simulink model "mixer_test"  (Simulink 7.0)
settings: Solver=VariableStepDiscrete  StartTime=0.0  StopTime=1500  RelTol=1e-3
libraries: xbsIndex_r4 x28, simulink x8, casper_library x6
settings Model: Creator=User  LastModifiedBy=User

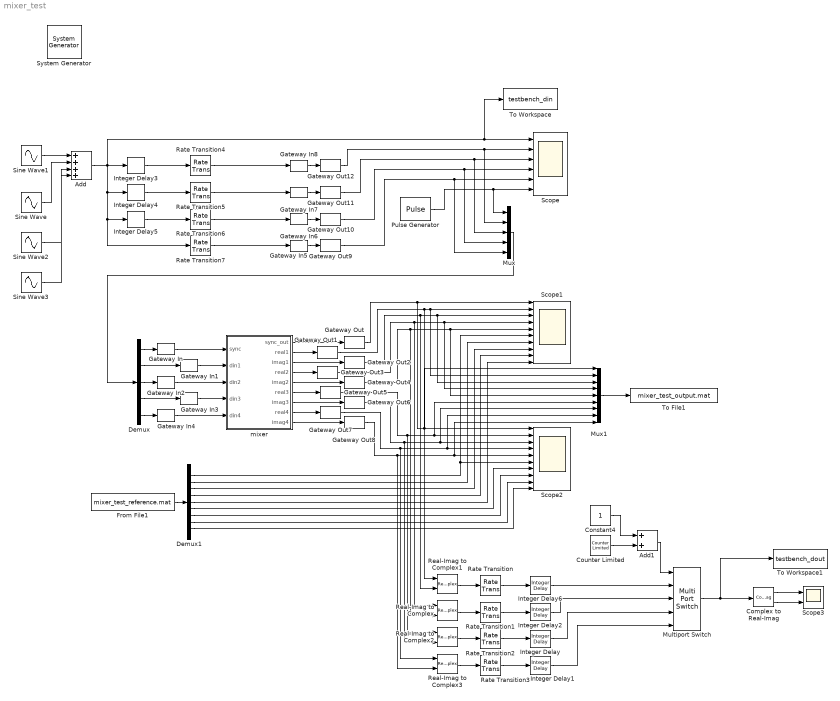
== system mixer_test ==
  " System Generator" : xbsIndex_r4/ System Generator  Tag=genX  SystemSampleTime=-1  xilinxfamily=Virtex4  part=xc4vsx35  speed=-10  package=ff668  synthesis_tool=XST  clock_wrapper=Clock Enables  directory=./netlist  testbench=off  simulink_period=1  sysclk_period=100  dcm_input_clock_period=100  incr_netlist=off  trim_vbits=Everywhere in SubSystem  dbl_ovrd=According to Block Masks  core_generation=According to Block Masks  run_coregen=off  deprecated_control=off  eval_field=0  block_type=sysgen
      settings: block_version=10.1.1
  Add : Sum  Inputs=++++  OutDataType=sfix(16)  OutScaling=2^-10
  Add1 : Sum  OutDataType=sfix(16)  OutScaling=2^-10
  Complex to Real-Imag : ComplexToRealImag
  Constant4 : Constant  OutDataType=sfix(16)  OutScaling=2^0
  Counter Limited : simulink/Sources/Counter Limited  SystemSampleTime=-1  uplimit=3  tsamp=-1
  Demux : Demux  Outputs=5
  Demux1 : Demux  Outputs=9
  From File1 : FromFile  FileName=mixer_test_reference.mat  SampleTime=1
  Gateway In : xbsIndex_r4/Gateway In  arith_type=Boolean  n_bits=16  bin_pt=14  quantization="Round  (unbiased: +/- Inf)"  overflow=Saturate  period=1  dbl_ovrd=off  timing_constraint=None  locs_specified=off  LOCs={}  block_type=gatewayin
      settings: infoedit="Gateway in block.  Converts inputs of type Simulink integer, double and fixed point to  Xilinx fixed point type.<P><P>Hardware notes:  In hardware these blocks become top level input ports."  block_version=10.1.1
  Gateway In{1..4,8} (5 alike) : xbsIndex_r4/Gateway In  arith_type="Signed  (2's comp)"  n_bits=16  bin_pt=13  quantization=Truncate  overflow=Wrap  period=1  dbl_ovrd=off  timing_constraint=None  locs_specified=off  LOCs={}  block_type=gatewayin
      settings: infoedit="Gateway in block.  Converts inputs of type Simulink integer, double and fixed point to  Xilinx fixed point type.<P><P>Hardware notes:  In hardware these blocks become top level input ports."  block_version=10.1.1
  Gateway In5 : xbsIndex_r4/Gateway In  arith_type="Signed  (2's comp)"  n_bits=16  bin_pt=13  quantization="Round  (unbiased: +/- Inf)"  overflow=Saturate  period=1  dbl_ovrd=off  timing_constraint=None  locs_specified=off  LOCs={}  block_type=gatewayin
      settings: infoedit="Gateway in block.  Converts inputs of type Simulink integer, double and fixed point to  Xilinx fixed point type.<P><P>Hardware notes:  In hardware these blocks become top level input ports."  block_version=10.1.1
  Gateway In6 : xbsIndex_r4/Gateway In  arith_type="Signed  (2's comp)"  n_bits=16  bin_pt=13  quantization="Round  (unbiased: +/- Inf)"  overflow=Saturate  period=1  dbl_ovrd=off  timing_constraint=None  locs_specified=off  LOCs={}  block_type=gatewayin
      settings: infoedit="Gateway in block.  Converts inputs of type Simulink integer, double and fixed point to  Xilinx fixed point type.<P><P>Hardware notes:  In hardware these blocks become top level input ports."  block_version=10.1.1
  Gateway In7 : xbsIndex_r4/Gateway In  arith_type="Signed  (2's comp)"  n_bits=16  bin_pt=13  quantization="Round  (unbiased: +/- Inf)"  overflow=Saturate  period=1  dbl_ovrd=off  timing_constraint=None  locs_specified=off  LOCs={}  block_type=gatewayin
      settings: infoedit="Gateway in block.  Converts inputs of type Simulink integer, double and fixed point to  Xilinx fixed point type.<P><P>Hardware notes:  In hardware these blocks become top level input ports."  block_version=10.1.1
  Gateway Out{,1..12} (13 alike) : xbsIndex_r4/Gateway Out  hdl_port=on  timing_constraint=None  locs_specified=off  LOCs={}  block_type=gatewayout
      settings: infoedit="Gateway out block.  Converts Xilinx fixed point inputs into ouputs of type Simulink integer, double, or fixed point.<P><P>Hardware notes:  In hardware these blocks become top level output ports or are discarded, depending on how they are configured."  block_version=10.1.1
  Integer Delay : simulink/Discrete/Integer Delay  vinit=0.0  samptime=0.25  NumDelays=3
  Integer Delay1 : simulink/Discrete/Integer Delay  vinit=0.0  samptime=0.25  NumDelays=4
  Integer Delay2 : simulink/Discrete/Integer Delay  vinit=0.0  samptime=0.25  NumDelays=2
  Integer Delay3 : simulink/Discrete/Integer Delay  vinit=0.0  samptime=-1  NumDelays=3
  Integer Delay4 : simulink/Discrete/Integer Delay  vinit=0.0  samptime=-1  NumDelays=2
  Integer Delay5 : simulink/Discrete/Integer Delay  vinit=0.0  samptime=-1  NumDelays=1
  Integer Delay6 : simulink/Discrete/Integer Delay  vinit=0.0  samptime=0.25  NumDelays=1
  Multiport Switch : MultiPortSwitch  OutDataType=sfix(16)  OutScaling=2^0
  Mux : Mux  Inputs=5
  Mux1 : Mux  Inputs=9
  Pulse Generator : DiscretePulseGenerator  Period=128  PhaseDelay=15
  Rate Transition{,1..7} (8 alike) : RateTransition
  Real-Imag to Complex{,1..3} (4 alike) : RealImagToComplex
  Scope : Scope  NumInputPorts=6
      settings: YMin=-5~-5~-5~-5~-5~-5  YMax=5~5~5~5~5~5
  Scope1 : Scope  NumInputPorts=10
      settings: YMin=-5~-5~-5~-5~-5~-5~-5~-5~-5~-5  YMax=5~5~5~5~5~5~5~5~5~5
  Scope2 : Scope  NumInputPorts=10
      settings: YMin=-5~-5~-5~-5~-5~-5~-5~-5~-5~-5  YMax=5~5~5~5~5~5~5~5~5~5  SaveName=ScopeData2
  Scope3 : Scope  NumInputPorts=2
      settings: YMin=-5~-5  YMax=5~5  SaveName=ScopeData3
  Sine Wave : Sin  SineType=Sample based  Samples=4  SampleTime=0.25
  Sine Wave1 : Sin  SineType=Sample based  Samples=3  SampleTime=0.25
  Sine Wave2 : Sin  SineType=Sample based  Samples=8  SampleTime=0.25
  Sine Wave3 : Sin  SineType=Sample based  Samples=16  SampleTime=0.25
  To File1 : ToFile  Filename=mixer_test_output.mat  MatrixName=output
  To Workspace : ToWorkspace  VariableName=testbench_din  SampleTime=-1  SaveFormat=Array
  To Workspace1 : ToWorkspace  VariableName=testbench_dout  SampleTime=-1  SaveFormat=Array
  mixer : Subsystem  AncestorBlock=casper_library/Downconverter/mixer  mask(mixer){freq_div=8, freq=1, nstreams=4, n_bits=10, bram_latency=3, mult_latency=3}
      mask prompts: freq_div "Frequency Divisions (M)"; freq "Mixing Frequency (? / M*2pi)"; nstreams "Number of Parallel Streams"; n_bits "Bit Width"; bram_latency "BRAM Latency"; mult_latency "Mult Latency"
      mask help: Digitally mixes an input signal (which can be several samples in parallel) with an LO of the indicated frequency (which is some fraction of the native FPGA clock rate).
      mask init:
      | mixer_init(gcb, ...
      |     'freq_div', freq_div, ...
      |     'freq', freq, ...
      |     'nstreams', nstreams, ...
      |     'n_bits', n_bits, ...
      |     'bram_latency', bram_latency, ...
      |     'mult_latency', mult_latency);
      settings: AttributesFormatString=lo at -1/8
      mask Help: eval('xlWeb([getenv(''MLIB_ROOT''), ''\doc\htmlblocks\sp_mixer\sp_mixer.html''])')
  wires:
  Mux/1 -> Demux/1
  Demux/1 -> Gateway In/1
  Demux/2 -> Gateway In1/1
  Demux/3 -> Gateway In2/1
  Demux/4 -> Gateway In3/1
  Demux/5 -> Gateway In4/1
  mixer/1(sync_out) -> Gateway Out/1
  mixer/2(real1) -> Gateway Out1/1
  mixer/3(imag1) -> Gateway Out2/1
  mixer/4(real2) -> Gateway Out3/1
  mixer/5(imag2) -> Gateway Out4/1
  mixer/6(real3) -> Gateway Out5/1
  mixer/7(imag3) -> Gateway Out6/1
  mixer/8(real4) -> Gateway Out7/1
  mixer/9(imag4) -> Gateway Out8/1
  Pulse Generator/1 -> Mux/1, Scope/6
  Gateway In/1 -> mixer/1(sync)
  Gateway In1/1 -> mixer/2(din1)
  Gateway In2/1 -> mixer/3(din2)
  Gateway In3/1 -> mixer/4(din3)
  Gateway In4/1 -> mixer/5(din4)
  Gateway Out/1 -> Scope1/1, Scope2/1, Mux1/1
  Gateway Out1/1 -> Scope1/2, Mux1/2, Real-Imag to Complex1/1
  Gateway Out3/1 -> Scope1/4, Mux1/4, Real-Imag to Complex/1
  Gateway Out4/1 -> Scope1/5, Mux1/5, Real-Imag to Complex/2
  Gateway Out5/1 -> Scope2/2, Mux1/6, Real-Imag to Complex2/1
  Gateway Out6/1 -> Scope2/3, Mux1/7, Real-Imag to Complex2/2
  Gateway Out7/1 -> Scope2/4, Mux1/8, Real-Imag to Complex3/1
  Gateway Out8/1 -> Scope2/5, Mux1/9, Real-Imag to Complex3/2
  Gateway In5/1 -> Gateway Out9/1
  Gateway Out9/1 -> Mux/5, Scope/5
  Gateway In8/1 -> Gateway Out12/1
  Gateway Out12/1 -> Mux/2, Scope/2
  Gateway In7/1 -> Gateway Out11/1
  Gateway Out11/1 -> Mux/3, Scope/3
  Gateway In6/1 -> Gateway Out10/1
  Gateway Out10/1 -> Mux/4, Scope/4
  Gateway Out2/1 -> Scope1/3, Mux1/3, Real-Imag to Complex1/2
  Mux1/1 -> To File1/1
  From File1/1 -> Demux1/1
  Demux1/1 -> Scope2/6, Scope1/6
  Demux1/2 -> Scope1/7
  Demux1/3 -> Scope1/8
  Demux1/4 -> Scope1/9
  Demux1/5 -> Scope1/10
  Demux1/6 -> Scope2/7
  Demux1/7 -> Scope2/8
  Demux1/8 -> Scope2/9
  Demux1/9 -> Scope2/10
  Complex to Real-Imag/1 -> Scope3/1
  Complex to Real-Imag/2 -> Scope3/2
  Add/1 -> Integer Delay5/1, Rate Transition7/1, Integer Delay4/1, Integer Delay3/1, To Workspace/1, Scope/1
  Integer Delay3/1 -> Rate Transition4/1
  Integer Delay4/1 -> Rate Transition5/1
  Integer Delay5/1 -> Rate Transition6/1
  Constant4/1 -> Add1/1
  Counter Limited/1 -> Add1/2
  Add1/1 -> Multiport Switch/1
  Real-Imag to Complex1/1 -> Rate Transition/1
  Real-Imag to Complex/1 -> Rate Transition1/1
  Real-Imag to Complex2/1 -> Rate Transition2/1
  Real-Imag to Complex3/1 -> Rate Transition3/1
  Multiport Switch/1 -> Complex to Real-Imag/1, To Workspace1/1
  Integer Delay1/1 -> Multiport Switch/5
  Integer Delay/1 -> Multiport Switch/4
  Integer Delay2/1 -> Multiport Switch/3
  Integer Delay6/1 -> Multiport Switch/2
  Rate Transition/1 -> Integer Delay6/1
  Rate Transition1/1 -> Integer Delay2/1
  Rate Transition2/1 -> Integer Delay/1
  Rate Transition3/1 -> Integer Delay1/1
  Rate Transition4/1 -> Gateway In8/1
  Rate Transition5/1 -> Gateway In7/1
  Rate Transition6/1 -> Gateway In6/1
  Rate Transition7/1 -> Gateway In5/1
  Sine Wave1/1 -> Add/1
  Sine Wave/1 -> Add/2
  Sine Wave2/1 -> Add/3
  Sine Wave3/1 -> Add/4

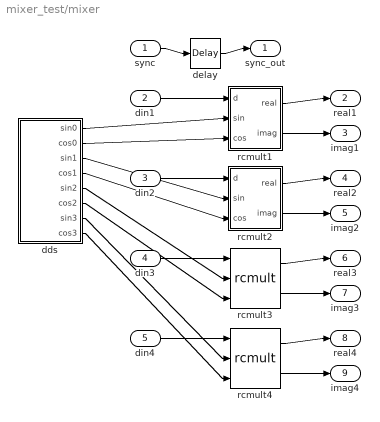
== system mixer_test/mixer ==
  sync : Inport  OutDataType=sfix(16)  OutScaling=2^0
  din1 : Inport  Port=2  OutDataType=sfix(16)  OutScaling=2^0
  din2 : Inport  Port=3  OutDataType=sfix(16)  OutScaling=2^0
  din3 : Inport  Port=4
  din4 : Inport  Port=5
  dds : Subsystem  AncestorBlock=casper_library/Downconverter/dds  mask(dds){freq_div=8, freq=1, num_lo=4, n_bits=10, latency=2}
      mask prompts: freq_div "Frequency divisions (M)"; freq "Frequency (? / M*2pi)"; num_lo "Parallel LOs"; n_bits "Bit Width"
      mask init:
      | dds_init(gcb, ...
      |     'freq_div', freq_div, ...
      |     'freq', freq, ...
      |     'num_lo', num_lo, ...
      |     'n_bits', n_bits, ...
      |     'latency', latency);
      settings: AttributesFormatString=lo at -1/8
  delay : xbsIndex_r4/Delay  en=off  latency=3  dbl_ovrd=off  reg_retiming=off  block_type=delay
      settings: xl_area=[0, 0, 0, 0, 0, 0, 0]  block_version=9.1.01
  rcmult1 : Subsystem  AncestorBlock=casper_library/Downconverter/rcmult  mask(rcmult){latency=3}
  rcmult2 : Subsystem  AncestorBlock=casper_library/Downconverter/rcmult  mask(rcmult){latency=3}
  rcmult3 : casper_library/Downconverter/rcmult  SystemSampleTime=-1  latency=3
  rcmult4 : casper_library/Downconverter/rcmult  SystemSampleTime=-1  latency=3
  sync_out : Outport  OutDataType=sfix(16)  OutScaling=2^0
  real1 : Outport  Port=2  OutDataType=sfix(16)  OutScaling=2^0
  imag1 : Outport  Port=3  OutDataType=sfix(16)  OutScaling=2^0
  real2 : Outport  Port=4  OutDataType=sfix(16)  OutScaling=2^0
  imag2 : Outport  Port=5  OutDataType=sfix(16)  OutScaling=2^0
  real3 : Outport  Port=6
  imag3 : Outport  Port=7
  real4 : Outport  Port=8
  imag4 : Outport  Port=9
  wires:
  rcmult4/2 -> imag4/1
  rcmult4/1 -> real4/1
  dds/8(cos3) -> rcmult4/3
  dds/7(sin3) -> rcmult4/2
  din4/1 -> rcmult4/1
  rcmult3/2 -> imag3/1
  rcmult3/1 -> real3/1
  dds/6(cos2) -> rcmult3/3
  dds/5(sin2) -> rcmult3/2
  din3/1 -> rcmult3/1
  rcmult2/2(imag) -> imag2/1
  rcmult2/1(real) -> real2/1
  dds/4(cos1) -> rcmult2/3(cos)
  dds/3(sin1) -> rcmult2/2(sin)
  din2/1 -> rcmult2/1(d)
  rcmult1/2(imag) -> imag1/1
  rcmult1/1(real) -> real1/1
  dds/2(cos0) -> rcmult1/3(cos)
  dds/1(sin0) -> rcmult1/2(sin)
  din1/1 -> rcmult1/1(d)
  delay/1 -> sync_out/1
  sync/1 -> delay/1

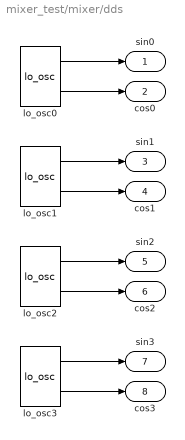
== system mixer_test/mixer/dds ==
  lo_osc0 : casper_library/Downconverter/lo_osc  SystemSampleTime=-1  n_bits=10  counter_step=4  counter_start=0  counter_width=3  latency=2
      link override counter: start_count=counter_start  cnt_by_val=counter_step  n_bits=counter_width
  lo_osc1 : casper_library/Downconverter/lo_osc  SystemSampleTime=-1  n_bits=10  counter_step=4  counter_start=1  counter_width=3  latency=2
      link override counter: start_count=counter_start  cnt_by_val=counter_step  n_bits=counter_width
  lo_osc2 : casper_library/Downconverter/lo_osc  SystemSampleTime=-1  n_bits=10  counter_step=4  counter_start=2  counter_width=3  latency=2
      link override counter: start_count=counter_start  cnt_by_val=counter_step  n_bits=counter_width
  lo_osc3 : casper_library/Downconverter/lo_osc  SystemSampleTime=-1  n_bits=10  counter_step=4  counter_start=3  counter_width=3  latency=2
      link override counter: start_count=counter_start  cnt_by_val=counter_step  n_bits=counter_width
  sin0 : Outport  OutDataType=sfix(16)  OutScaling=2^0
  cos0 : Outport  Port=2  OutDataType=sfix(16)  OutScaling=2^0
  sin1 : Outport  Port=3  OutDataType=sfix(16)  OutScaling=2^0
  cos1 : Outport  Port=4  OutDataType=sfix(16)  OutScaling=2^0
  sin2 : Outport  Port=5
  cos2 : Outport  Port=6
  sin3 : Outport  Port=7
  cos3 : Outport  Port=8
  wires:
  lo_osc3/2 -> cos3/1
  lo_osc3/1 -> sin3/1
  lo_osc2/2 -> cos2/1
  lo_osc2/1 -> sin2/1
  lo_osc1/2 -> cos1/1
  lo_osc1/1 -> sin1/1
  lo_osc0/2 -> cos0/1
  lo_osc0/1 -> sin0/1

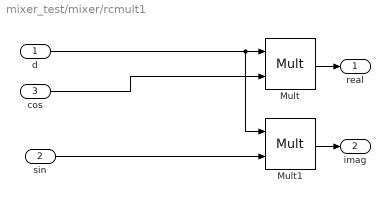
== system mixer_test/mixer/rcmult1 ==
  d : Inport  OutDataType=sfix(16)  OutScaling=2^0
  sin : Inport  Port=2  OutDataType=sfix(16)  OutScaling=2^0
  cos : Inport  Port=3  OutDataType=sfix(16)  OutScaling=2^0
  Mult : xbsIndex_r4/Mult  precision=Full  arith_type="Signed  (2's comp)"  n_bits=8  bin_pt=2  quantization=Truncate  overflow=Wrap  en=off  latency=latency  dbl_ovrd=off  use_behavioral_HDL=off  use_embedded=on  opt=Speed  optimum_pipeline=off  pipeline=on  use_rpm=off  placement_style=Rectangular shape  block_type=mult
      settings: infoedit=Hardware notes: To use the internal pipeline stage of the dedicated multiplier you must select 'Pipeline for maximum performance'.  xl_area=[0, 0, 0, 0, 0, 0, 0]  block_version=9.1.01
  Mult1 : xbsIndex_r4/Mult  precision=Full  arith_type="Signed  (2's comp)"  n_bits=8  bin_pt=2  quantization=Truncate  overflow=Wrap  en=off  latency=latency  dbl_ovrd=off  use_behavioral_HDL=off  use_embedded=on  opt=Speed  optimum_pipeline=off  pipeline=on  use_rpm=off  placement_style=Rectangular shape  block_type=mult
      settings: infoedit=Hardware notes: To use the internal pipeline stage of the dedicated multiplier you must select 'Pipeline for maximum performance'.  xl_area=[0, 0, 0, 0, 0, 0, 0]  block_version=9.1.01
  real : Outport  OutDataType=sfix(16)  OutScaling=2^0
  imag : Outport  Port=2  OutDataType=sfix(16)  OutScaling=2^0
  wires:
  cos/1 -> Mult/2
  sin/1 -> Mult1/2
  d/1 -> Mult/1, Mult1/1
  Mult/1 -> real/1
  Mult1/1 -> imag/1

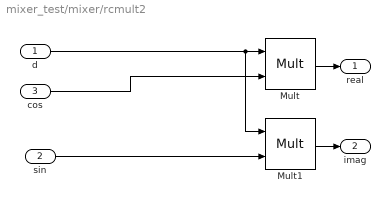
== system mixer_test/mixer/rcmult2 ==
  d : Inport  OutDataType=sfix(16)  OutScaling=2^0
  sin : Inport  Port=2  OutDataType=sfix(16)  OutScaling=2^0
  cos : Inport  Port=3  OutDataType=sfix(16)  OutScaling=2^0
  Mult : xbsIndex_r4/Mult  precision=Full  arith_type="Signed  (2's comp)"  n_bits=8  bin_pt=2  quantization=Truncate  overflow=Wrap  en=off  latency=latency  dbl_ovrd=off  use_behavioral_HDL=off  use_embedded=on  opt=Speed  optimum_pipeline=off  pipeline=on  use_rpm=off  placement_style=Rectangular shape  block_type=mult
      settings: infoedit=Hardware notes: To use the internal pipeline stage of the dedicated multiplier you must select 'Pipeline for maximum performance'.  xl_area=[0, 0, 0, 0, 0, 0, 0]  block_version=9.1.01
  Mult1 : xbsIndex_r4/Mult  precision=Full  arith_type="Signed  (2's comp)"  n_bits=8  bin_pt=2  quantization=Truncate  overflow=Wrap  en=off  latency=latency  dbl_ovrd=off  use_behavioral_HDL=off  use_embedded=on  opt=Speed  optimum_pipeline=off  pipeline=on  use_rpm=off  placement_style=Rectangular shape  block_type=mult
      settings: infoedit=Hardware notes: To use the internal pipeline stage of the dedicated multiplier you must select 'Pipeline for maximum performance'.  xl_area=[0, 0, 0, 0, 0, 0, 0]  block_version=9.1.01
  real : Outport  OutDataType=sfix(16)  OutScaling=2^0
  imag : Outport  Port=2  OutDataType=sfix(16)  OutScaling=2^0
  wires:
  cos/1 -> Mult/2
  sin/1 -> Mult1/2
  d/1 -> Mult/1, Mult1/1
  Mult/1 -> real/1
  Mult1/1 -> imag/1
